simulink model "RSTcommand"  (R2021a)
settings: Solver=VariableStepAuto  StartTime=0.0  StopTime=10  RelTol=1e-3
undefined symbols (not defined in the file or in its folder): filt
libraries: cstblocks x3
settings Model: Creator=alaba  LastModifiedBy=alaba

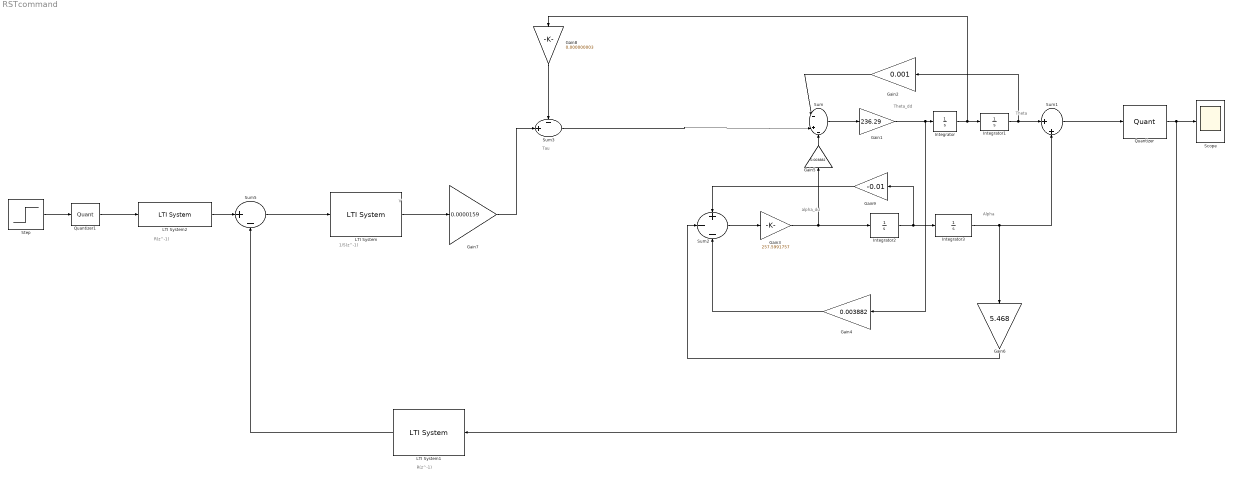
== system RSTcommand ==
  note: R(z^-1)
  note: Theta
  note: Alpha
  note: alpha_dd
  note: Theta_dd
  note: Tau
  note: V
  note: R(z^-1)
  note: 1/S(z^-1)
  Gain1 : Gain  Gain=236.29
  Gain2 : Gain  Gain=0.001
  Gain3 : Gain  Gain=257.5991757
  Gain4 : Gain  Gain=0.003882
  Gain5 : Gain  Gain=0.003882
  Gain6 : Gain  Gain=5.468
  Gain7 : Gain  Gain=0.0000159
  Gain8 : Gain  Gain=0.000000003
  Gain9 : Gain  Gain=-0.01
  Integrator{,1..3} (4 alike) : Integrator
  LTI System : cstblocks/LTI System  sys=filt(1,[1 -0.1725 -1.9682 1.1814 ])  IC=[]
  LTI System1 : cstblocks/LTI System  sys=filt([465.8971 -971.1233 491.0839 -0.0097],[1])  IC=[]
  LTI System2 : cstblocks/LTI System  sys=filt([465.8971 -971.1233 491.0839 -0.0097],[1])  IC=[]
  Quantizer : Quantizer  QuantizationInterval=0.1
  Quantizer1 : Quantizer  QuantizationInterval=0.1
  Scope : Scope
  Step : Step  Time=0.1  Before=1  After=100  SampleTime=0.1
  Sum : Sum  Inputs=|-+-
  Sum1 : Sum  Inputs=|++
  Sum2 : Sum  Inputs=+--
  Sum3 : Sum  Inputs=-+|
  Sum5 : Sum  Inputs=|+-
  wires:
  Integrator/1 -> Integrator1/1, Gain8/1
  Integrator2/1 -> Gain9/1, Integrator3/1
  Sum/1 -> Gain1/1
  Gain1/1 -> Gain4/1, Integrator/1
  Integrator3/1 -> Sum1/2, Gain6/1
  Integrator1/1 -> Sum1/1, Gain2/1
  Gain3/1 -> Integrator2/1, Gain5/1
  Sum2/1 -> Gain3/1
  Gain5/1 -> Sum/3
  Gain7/1 -> Sum3/2
  Gain8/1 -> Sum3/1
  Sum3/1 -> Sum/2
  Gain2/1 -> Sum/1
  Gain4/1 -> Sum2/3
  Gain6/1 -> Sum2/2
  Gain9/1 -> Sum2/1
  Quantizer1/1 -> LTI System2/1
  LTI System/1 -> Gain7/1
  Quantizer/1 -> LTI System1/1, Scope/1
  LTI System1/1 -> Sum5/2
  LTI System2/1 -> Sum5/1
  Sum1/1 -> Quantizer/1
  Sum5/1 -> LTI System/1
  Step/1 -> Quantizer1/1
